simulink model "finite_state_machines"  (R2020a)
settings: Solver=VariableStepAuto  StartTime=0.0  StopTime=20.0  RelTol=1e-3
settings Model: Creator=Callum  LastModifiedBy=Callum

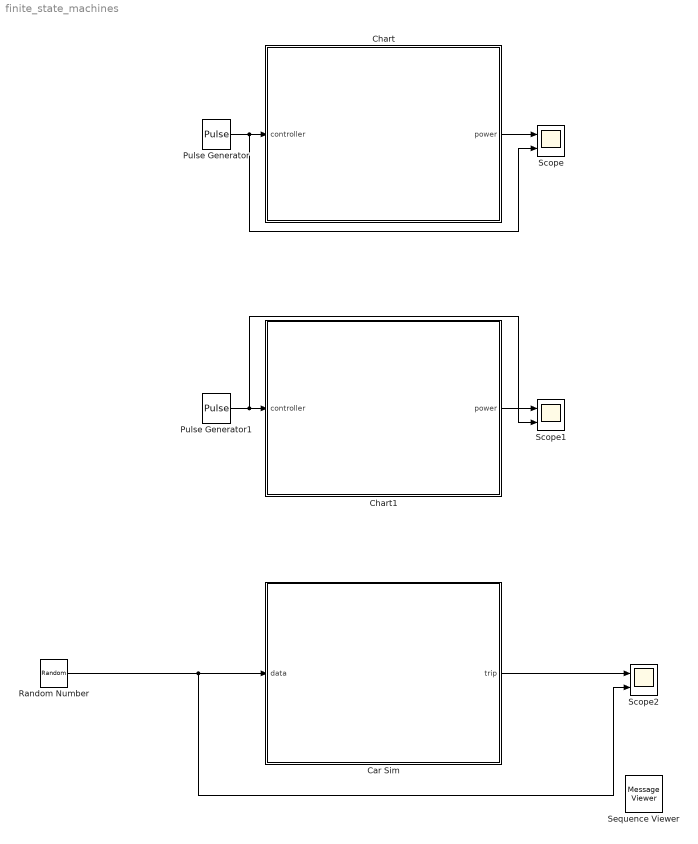
== system finite_state_machines ==
  Car Sim : Stateflow chart  TreatAsAtomicUnit=on
  Chart : Stateflow chart  TreatAsAtomicUnit=on
  Chart1 : Stateflow chart  TreatAsAtomicUnit=on
  Pulse Generator : DiscretePulseGenerator  PulseType=Time based  Period=1  PulseWidth=5
  Pulse Generator1 : DiscretePulseGenerator  PulseType=Time based  Period=1  PulseWidth=5
  Random Number : RandomNumber  Mean=280  Variance=150  SampleTime=0.1
  Scope : Scope  NumInputPorts=2
  Scope1 : Scope  NumInputPorts=2
  Scope2 : Scope  NumInputPorts=2
  Sequence Viewer : MessageViewer  History=1000  SavedRootId=#
  wires:
  Chart1/1(power) -> Scope1/1
  Chart/1(power) -> Scope/1
  Pulse Generator1/1 -> Chart1/1(controller), Scope1/2
  Pulse Generator/1 -> Scope/2, Chart/1(controller)
  Random Number/1 -> Scope2/2, Car Sim/1(data)
  Car Sim/1(trip) -> Scope2/1

== stateflow chart finite_state_machines/Chart1 ==
  state power_off
    en:
    power=0;
  state power_on
    en:
    power=1;
  (default) -> power_off
  power_off -> power_on : [controller == 1]
  power_on -> power_off : after(0.5, sec)
  data: controller input; power output

== stateflow chart finite_state_machines/Car Sim ==
  state driver [parallel]
    settings: executionOrder=1
    state waiting_in_parking
    state driving
      trip = trip - x
    state reaching_destination
    (default) -> waiting_in_parking
    waiting_in_parking -> driving : [data > 300]
        | {
        | send(sth_happened, car);
        | trip=data;
        | }
    reaching_destination -> waiting_in_parking : [x == 0]
    driving -> driving [order 2] : after(1, sec)
    driving -> reaching_destination [order 1] : [trip <= 0]
        | {
        | send(dest_reached, car)
        | }
  state car [parallel]
    settings: executionOrder=2
    state idle
      x = 0
    state decceleration
      x = x - 1
    state acceleration
      x = x + 1
    state cruising
    (default) -> idle
    idle -> acceleration : sth_happened
    (junction 25) -> idle [order 1] : [x <= 0]
    (junction 25) -> decceleration [order 2]
    decceleration -> (junction 25) : after(1, sec)
    (junction 20) -> acceleration [order 2]
    cruising -> decceleration : dest_reached
    acceleration -> (junction 20) : after(1, sec)
    (junction 20) -> cruising [order 1] : [x >= 10]
  data: trip output; data input; x local
  events: sth_happened local FUNCTION_CALL_EVENT; dest_reached local FUNCTION_CALL_EVENT

== stateflow chart finite_state_machines/Chart ==
  state init
  state power_off
    en:
    power=0;
  state power_on
    en:
    power=1;
  (default) -> init : {power=0}
  power_off -> init
  init -> power_on : [controller == 1]
  power_on -> power_off : after(0.5, sec)
  data: controller input; power output
